simulink model "navigateObstacle_SF_solution"  (R2022a)
settings: Solver=ode23t  StartTime=0.0  StopTime=inf  RelTol=1e-3
InitFcn:
  | RPInit
model workspace (MAT data in the model file):
  mapForSim.obsMap = [0 0 0 0 0 0 0 0 0 0 0 0 ... (26600 elements, 133x200)]
  mapForSim.scaleFactor = 33.3333333333
  mapForSim.simMap = robotics.BinaryOccupancyGrid
  mapForSim.simMap.Grid = [1 1 1 1 1 1 1 1 1 1 1 1 ... (26600 elements, 133x200)]
  mapForSim.simMap.SharedProperties = matlabshared.autonomous.internal.SharedMapProperties
  mapForSim.simMap.SharedProperties.Resolution = 33.3333333333
  mapForSim.simMap.SharedProperties.GridSize = [133 200]
  mapForSim.simMap.SharedProperties.XLocalLimits = [0 6]
  mapForSim.simMap.SharedProperties.YLocalLimits = [0 3.99]
  mapForSim.simMap.SharedProperties.XWorldLimits = [0 6]
  mapForSim.simMap.SharedProperties.YWorldLimits = [0 3.99]
  mapForSim.simMap.SharedProperties.Width = 6
  mapForSim.simMap.SharedProperties.Height = 3.99
  mapForSim.simMap.SharedProperties.LocalOriginInWorldInternal = [0 0]
  mapForSim.simMap.LayerName = 'binaryLayer'
  mapForSim.simMap.Index = matlabshared.autonomous.internal.CircularBufferIndex
  mapForSim.simMap.Index.Head = [1 1]
  mapForSim.simMap.Index.Size = [133 200]
  mapForSim.simMap.Index.NewRegions = [0 0 0 0]
  mapForSim.simMap.Index.DropEntireMap = 0
  mapForSim.simMap.Index.DropTwoRegions = [0 0]
  mapForSim.simMap.Buffer = matlabshared.autonomous.internal.CircularBuffer
  mapForSim.simMap.Buffer.ConstVal = 0
  mapForSim.simMap.Buffer.DataType = 'logical'
  mapForSim.simMap.Buffer.Index = matlabshared.autonomous.internal.CircularBufferIndex
  mapForSim.simMap.Buffer.Index.Head = [1 1]
  mapForSim.simMap.Buffer.Index.Size = [133 200]
  mapForSim.simMap.Buffer.Index.NewRegions = [0 0 0 0]
  mapForSim.simMap.Buffer.Index.DropEntireMap = 0
  mapForSim.simMap.Buffer.Index.DropTwoRegions = [0 0]
  mapForSim.simMap.Buffer.Buffer = [1 1 1 1 1 1 1 1 1 1 1 1 ... (26600 elements, 133x200)]
  mapForSim.simMap.Buffer.BufferSize = [133 200 1]
  mapForSim.simMap.DefaultValueInternal = 0
  mapForSim.simMap.DataSize = [133 200]
  mapForSim.simMap.GridLocationInWorld = [0 0]
  mapForSim.simMap.GridOriginInLocal = [0 0]
  mapForSim.simMap.LocalOriginInWorld = [0 0]
  mapForSim.simMap.Resolution = 33.3333333333
  mapForSim.simMap.GridSize = [133 200]
  mapForSim.simMap.XLocalLimits = [0 6]
  mapForSim.simMap.YLocalLimits = [0 3.99]
  mapForSim.simMap.XWorldLimits = [0 6]
  mapForSim.simMap.YWorldLimits = [0 3.99]
  occGrid = robotics.BinaryOccupancyGrid
  occGrid.Grid = [1 1 1 1 1 1 1 1 1 1 1 1 ... (26600 elements, 133x200)]
  occGrid.SharedProperties = matlabshared.autonomous.internal.SharedMapProperties
  occGrid.SharedProperties.Resolution = 33.3333333333
  occGrid.SharedProperties.GridSize = [133 200]
  occGrid.SharedProperties.XLocalLimits = [0 6]
  occGrid.SharedProperties.YLocalLimits = [0 3.99]
  occGrid.SharedProperties.XWorldLimits = [0 6]
  occGrid.SharedProperties.YWorldLimits = [0 3.99]
  occGrid.SharedProperties.Width = 6
  occGrid.SharedProperties.Height = 3.99
  occGrid.SharedProperties.LocalOriginInWorldInternal = [0 0]
  occGrid.LayerName = 'binaryLayer'
  occGrid.Index = matlabshared.autonomous.internal.CircularBufferIndex
  occGrid.Index.Head = [1 1]
  occGrid.Index.Size = [133 200]
  occGrid.Index.NewRegions = [0 0 0 0]
  occGrid.Index.DropEntireMap = 0
  occGrid.Index.DropTwoRegions = [0 0]
  occGrid.Buffer = matlabshared.autonomous.internal.CircularBuffer
  occGrid.Buffer.ConstVal = 0
  occGrid.Buffer.DataType = 'logical'
  occGrid.Buffer.Index = matlabshared.autonomous.internal.CircularBufferIndex
  occGrid.Buffer.Index.Head = [1 1]
  occGrid.Buffer.Index.Size = [133 200]
  occGrid.Buffer.Index.NewRegions = [0 0 0 0]
  occGrid.Buffer.Index.DropEntireMap = 0
  occGrid.Buffer.Index.DropTwoRegions = [0 0]
  occGrid.Buffer.Buffer = [1 1 1 1 1 1 1 1 1 1 1 1 ... (26600 elements, 133x200)]
  occGrid.Buffer.BufferSize = [133 200 1]
  occGrid.DefaultValueInternal = 0
  occGrid.DataSize = [133 200]
  occGrid.GridLocationInWorld = [0 0]
  occGrid.GridOriginInLocal = [0 0]
  occGrid.LocalOriginInWorld = [0 0]
  occGrid.Resolution = 33.3333333333
  occGrid.GridSize = [133 200]
  occGrid.XLocalLimits = [0 6]
  occGrid.YLocalLimits = [0 3.99]
  occGrid.XWorldLimits = [0 6]
  occGrid.YWorldLimits = [0 3.99]
undefined symbols (not defined in the file): FloorSurface, Ref, RobotSurface, X, Y, Z
libraries: sm_lib x21, RP_Simulator_Components x12, nesl_utility x11, RoboticsPlayground x2
settings Model: Creator=josea  LastModifiedBy=josea
settings SolverCC: AlgebraicLoopSolver=TrustRegion
settings DataIOCC: ReturnWorkspaceOutputs=off
settings DebuggingCC: UnconnectedInputMsg=warning  UnconnectedOutputMsg=warning  SFMachineParentedDataDiag=warning  ArithmeticOperatorsInVariantConditions=warning
settings SFSimCC: SimUseLocalCustomCode=off  CustomCodeUndefinedFunction=UseInterfaceOnly
settings RTWCC: RTWUseLocalCustomCode=off
settings DiagnosticsConfigSet: SimMechanicsRigidlyBoundBlock=none
settings ExplorerConfigSet: InternalSimMechanicsExplorerSettings="<ExplorerConfiguration><canonicalview>default</canonicalview><AnimationSetting><BasePlaybackSpeed>1.0</BasePlaybackSpeed><PlaybackSpeedFactor>1.0</PlaybackSpeedFactor></AnimationSetting><TilePanel><TileInfo><Tiles Columns=\"1\" Count=\"1\" Rows=\"1\"><Column Weight=\"1\"/><Row Weight=\"1\"/><Tile Height=\"1\" Width=\"1\" X=\"0\" Y=\"0\"/></Tiles></TileInfo><SceneInfo><SceneViewer><BGColor><R>0.60000002384185791</R><G>0.60000002384185791</G><B>0.60000002384185791</B></BGColor><Camera><DoPerspective>off</DoPerspective><Position><X>1.02772841465426201</X><Y>-4.04307345472878321</Y><Z>5.44141009880599036</Z></Position><Center><X>1.02224964927968398</X><Y>0.073144029153633619</Y><Z>0.356451439525035663</Z></Center><Up><X>-0.0145298301603439817</X><Y>0.777168441982217129</Y><Z>0.629124865843375347</Z></Up><ViewLimDist>1</ViewLimDist><YLim>3.91326740754770297</YLim><XLim>6.08730485618531603</XLim></Camera></SceneViewer></SceneInfo></TilePanel><MechEditorPanel><Cameras/><GfxPanelCameraMap/><VideoCreator><PlaybackSpeedRatio>2.0</PlaybackSpeedRatio><FrameRate>30</FrameRate><VideoFormat>Motion JPEG AVI</VideoFormat><FrameSize>[1280 720]</FrameSize></VideoCreator></MechEditorPanel></ExplorerConfiguration>"

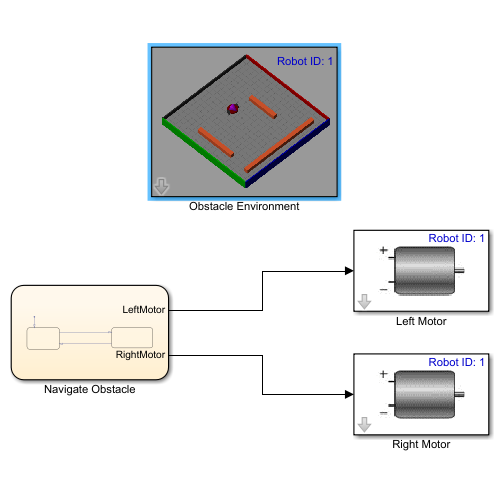
[thumbnail: Simulink's stored preview of the top-level diagram]
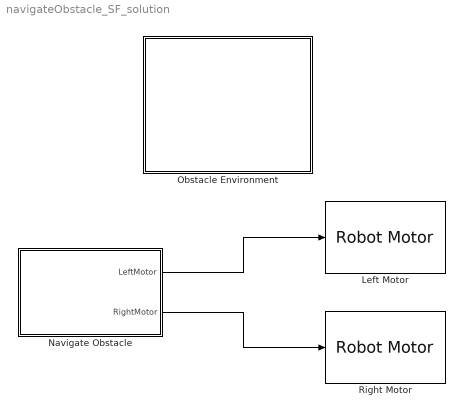
== system navigateObstacle_SF_solution ==
  Left Motor : RoboticsPlayground/Basic Sensors and Actuators/Robot Motor  robotId=1  motorChoice=1
      settings: SourceProductName=Robotics Playground
  Navigate Obstacle : Stateflow chart  TreatAsAtomicUnit=on
  Obstacle Environment : Subsystem  mask(RP Obstacle Environment){obs1=on, obsPose1=[0.054199    0.068864], obsWidth1=1.3052, obsLength1=1.156, obs2=off, obsPose2=[2.2548   -0.067351], obsWidth2=0.2899, obsLength2=3.4524, obs3=off, obsPose3=[-0.22694     -1.5652], obsWidth3=4.4627, obsLength3=0.4041, obs4=off, obsPose4=[-2.3001     0.17862], obsWidth4=0.4041, obsLength4=2.8726, obs5=off, obsPose5=[1.6535    -0.67545], obsWidth5=0.39824, obsLength5=0.71449, obs6=off, obsPose6=[3.1293     -1.6301], obsWidth6=0.60322, obsLength6=0.47438, obs7=off, obsPose7=[2 2], obsWidth7=0.8, obsLength7=0.4, obs8=off, obsPose8=[2 2], obsWidth8=0.8, obsLength8=0.4, obs9=off, obsPose9=[2 2], obsWidth9=0.8, obsLength9=0.4, obs10=off, obsPose10=[2 2], obsWidth10=0.8, obsLength10=0.4, arenaLength=6, arenaWidth=4, robotId=1, wheelBase=0.5, wheelRadius=0.1, robotColor=[0.5 0 0], startPose=[-1.2 -1.2]}
      mask prompts: obs1 "Enable"; obsPose1 "Position X Y [m]"; obsWidth1 "Width [m]"; obsLength1 "Length [m]"; obs2 "Enable"; obsPose2 "Position X Y [m]"; obsWidth2 "Width [m]"; obsLength2 "Length [m]"; obs3 "Enable"; obsPose3 "Position X Y [m]"; obsWidth3 "Width [m]"; obsLength3 "Length [m]"; obs4 "Enable"; obsPose4 "Position X Y [m]"; obsWidth4 "Width [m]"; obsLength4 "Length [m]"; obs5 "Enable"; obsPose5 "Position X Y [m]"; obsWidth5 "Width [m]"; obsLength5 "Length [m]"; obs6 "Enable"; obsPose6 "Position X Y [m]"; obsWidth6 "Width [m]"; obsLength6 "Length [m]"; obs7 "Enable"; obsPose7 "Position X Y [m]"; obsWidth7 "Width [m]"; obsLength7 "Length [m]"; obs8 "Enable"; obsPose8 "Position X Y [m]"; obsWidth8 "Width [m]"; obsLength8 "Length [m]"; obs9 "Enable"; obsPose9 "Position X Y [m]"; obsWidth9 "Width [m]"; obsLength9 "Length [m]"; obs10 "Enable"; obsPose10 "Position X Y [m]"; obsWidth10 "Width [m]"; obsLength10 "Length [m]"; arenaLength "Length [m]"; arenaWidth "Width [m]"; robotId "Robot ID"; wheelBase "Distance between wheels [m]"; wheelRadius "Wheel radius [m]"; robotColor "Color [R G B]"; startPose "Initial Position X Y [m]"
      mask help:
      | This block contains a virtual environment for a single robot to interact with walls, obstacles and objects. Sensors implemented in the Robotics Playground library can be used to obtain environment information and actuators to interact with the robot behavior.
      |
      | Motor mapping for the robot is as follows:
      |
      | Motor 1 -> Left wheel motor torque
      | Motor 2 -> Right wheel motor torque
      settings: CopyFcn=|
      | set_param(gcs,'InitFcn','RPInit');
      | set_param(gcs,'Solver','ode23t');
      | set_param(gcs, 'EnablePacing', 'on')
      | set_param(gcs, 'PacingRate', 1)
      mask Help: web('obstacle_arena.htm')
      mask Callback obs1: commentObstacles(gcb)
      mask Callback obs2: commentObstacles(gcb)
      mask Callback obs3: commentObstacles(gcb)
      mask Callback obs4: commentObstacles(gcb)
      mask Callback obs5: commentObstacles(gcb)
      mask Callback obs6: commentObstacles(gcb)
      mask Callback obs7: commentObstacles(gcb)
      mask Callback obs8: commentObstacles(gcb)
      mask Callback obs9: commentObstacles(gcb)
      mask Callback obs10: commentObstacles(gcb)
      mask DialogControl obsT Prompt: Obstacle settings
      mask DialogControl Container19 Prompt: Set Obstacles Interactively
      mask DialogControl Control2 Prompt: Set Obstacles
      mask DialogControl Control2 Callback: setObstaclesUI(gcb)
      mask DialogControl Control3 Prompt: Disable all obstacles
      mask DialogControl Control3 Callback: disableObstacles(gcb)
      mask DialogControl Container21 Prompt: Obstacle Details
      mask DialogControl obsc1 Prompt: Obstacle 1
      mask DialogControl obsc2 Prompt: Obstacle 2
      mask DialogControl obsc3 Prompt: Obstacle 3
      mask DialogControl obsc4 Prompt: Obstacle 4
      mask DialogControl obsc5 Prompt: Obstacle 5
      mask DialogControl obsc6 Prompt: Obstacle 6
      mask DialogControl obsc7 Prompt: Obstacle 7
      mask DialogControl obsc8 Prompt: Obstacle 8
      mask DialogControl obsc9 Prompt: Obstacle 9
      mask DialogControl obsc10 Prompt: Obstacle 10
      mask DialogControl Container6 Prompt: Arena settings
      mask DialogControl Container4 Prompt: Robot settings
      mask Display:
      | color('white');
      | plot([100,100,100,100]*1,[100,100,100,100]*1);
      | plot([100,100,100,100]*0,[100,100,100,100]*0);
      | image('ObstacleEnv.PNG')
      | color('blue');
      | id=eval(get_param(gcb,'robotId'));
      | text(99, 92, ['Robot ID: ' num2str(id)], 'horizontalAlignment', 'right');
  Right Motor : RoboticsPlayground/Basic Sensors and Actuators/Robot Motor  robotId=1  motorChoice=2
      settings: SourceProductName=Robotics Playground
  wires:
  Navigate Obstacle/1(LeftMotor) -> Left Motor/1
  Navigate Obstacle/2(RightMotor) -> Right Motor/1

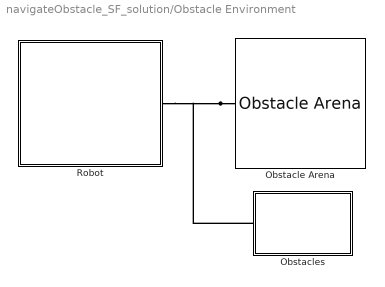
== system navigateObstacle_SF_solution/Obstacle Environment ==
  Obstacle Arena : RP_Simulator_Components/Obstacle Arena  length=arenaLength  width=arenaWidth  robotRadius=wheelBase/2
  Obstacles : Subsystem
  Robot : Subsystem  AncestorBlock=RP_Simulator_Components/Contact Tank Robot  mask(RP Contact Tank Robot){robotId=robotId, wheelRadius=wheelRadius, wheelBase=wheelBase, wheelThickness=0.025, chassisThickness=0.05, startPose=startPose, choice=off, sensorTs=0.05, wheelMass=0.2, chassisMass=0.5, maxWheelTorque=1, floorSize=[arenaLength arenaWidth], wheelColor=[0.25 0.25 0.25], chassisColor=robotColor}
      mask prompts: robotId "Robot ID"; wheelRadius "Wheel Radius [m]"; wheelBase "Wheelbase [m]"; wheelThickness "Wheel Thickness [m]"; chassisThickness "Chassis Thickness [m]"; startPose "Start Position [m]"; choice "Reverse Start Position"; sensorTs "Sensor sample time [s]"; wheelMass "Wheel Mass [kg]"; chassisMass "Chassis Mass [kg]"; maxWheelTorque "Maximum wheel torque [N*m]"; floorSize "Floor Dimensions [m]"; wheelColor "Wheel Color"; chassisColor "Chassis Color"
      mask help:
      | This robot implements contact between the robot wheels and the floor of an arena. The stck-slip friction implemented using contact force libraries makes the robot behavior more realistic. The inputs to the robot are now motor torque, which is set using the Robotics Playground Motor blocks. The motor mappings are as follows:
      |
      | Motor 1 -> Left wheel motor torque
      | Motor 2 -> Right wheel motor torque
      mask init:
      | block=gcb;
      | ID=num2str(eval(get_param(block,'robotId')));
      | 
      | set_param([block '/motor1t'],'GotoTag',['R' ID 'motor1t']);
      | set_param([block '/motor2t'],'GotoTag',['R' ID 'motor2t']);
      | set_param([block '/motor1q'],'GotoTag',['R' ID 'motor1q']);
      | set_param([block '/motor1w'],'GotoTag',['R' ID 'motor1w']);
      | set_param([block '/motor2q'],'GotoTag',['R' ID 'motor2q']);
      | set_param([block '/motor2w'],'GotoTag',['R' ID 'motor2w']);
      | set_param([block '/xPose'],'GotoTag',['R' ID 'xPose']);
      | set_param([block '/yPose'],'GotoTag',['R' ID 'yPose']);
      | set_param([block '/tPose'],'GotoTag',['R' ID 'tPose']);
      | set_param([block '/tRate'],'GotoTag',['R' ID 'tRate']);
      | set_param([block '/tAngle'],'GotoTag',['R' ID 'tAngle']);
      | 
      | % Add sensor visuals
      | 
      | addSensors(block,eval(ID));
      mask DialogControl KinContainer Prompt: Kinematics
      mask DialogControl DynamicsContainer Prompt: Dynamics
      mask DialogControl AppearanceContainer Prompt: Appearance
      mask Display:
      | image('discRobot.PNG')
      | port_label('Rconn',1,'RP-Bus')
  connections:
  Obstacle Arena/LConn1 -- Obstacles/LConn1 -- Robot/RConn1

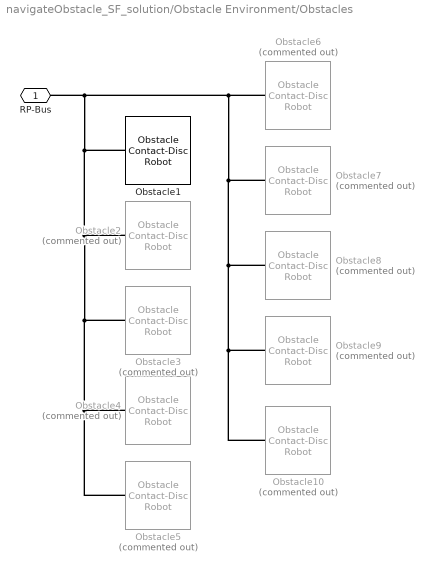
== system navigateObstacle_SF_solution/Obstacle Environment/Obstacles ==
  Obstacle1 : RP_Simulator_Components/Obstacle Contact-Disc Robot  Pose=obsPose1  width=obsWidth1  length=obsLength1  height=0.3  color=[1.0 0.4 0.2]
  Obstacle10 : RP_Simulator_Components/Obstacle Contact-Disc Robot  Commented=on  Pose=obsPose10  width=obsWidth10  length=obsLength10  height=0.3  color=[1.0 0.4 0.2]
  Obstacle2 : RP_Simulator_Components/Obstacle Contact-Disc Robot  Commented=on  Pose=obsPose2  width=obsWidth2  length=obsLength2  height=0.3  color=[1.0 0.4 0.2]
  Obstacle3 : RP_Simulator_Components/Obstacle Contact-Disc Robot  Commented=on  Pose=obsPose3  width=obsWidth3  length=obsLength3  height=0.3  color=[1.0 0.4 0.2]
  Obstacle4 : RP_Simulator_Components/Obstacle Contact-Disc Robot  Commented=on  Pose=obsPose4  width=obsWidth4  length=obsLength4  height=0.3  color=[1.0 0.4 0.2]
  Obstacle5 : RP_Simulator_Components/Obstacle Contact-Disc Robot  Commented=on  Pose=obsPose5  width=obsWidth5  length=obsLength5  height=0.3  color=[1.0 0.4 0.2]
  Obstacle6 : RP_Simulator_Components/Obstacle Contact-Disc Robot  Commented=on  Pose=obsPose6  width=obsWidth6  length=obsLength6  height=0.3  color=[1.0 0.4 0.2]
  Obstacle7 : RP_Simulator_Components/Obstacle Contact-Disc Robot  Commented=on  Pose=obsPose7  width=obsWidth7  length=obsLength7  height=0.3  color=[1.0 0.4 0.2]
  Obstacle8 : RP_Simulator_Components/Obstacle Contact-Disc Robot  Commented=on  Pose=obsPose8  width=obsWidth8  length=obsLength8  height=0.3  color=[1.0 0.4 0.2]
  Obstacle9 : RP_Simulator_Components/Obstacle Contact-Disc Robot  Commented=on  Pose=obsPose9  width=obsWidth9  length=obsLength9  height=0.3  color=[1.0 0.4 0.2]
  RP-Bus : PMIOPort  Side=Left
  connections:
  Obstacle1/LConn1 -- Obstacle5/LConn1 -- Obstacle4/LConn1 -- Obstacle3/LConn1 -- Obstacle2/LConn1 -- Obstacle6/LConn1 -- Obstacle10/LConn1 -- Obstacle9/LConn1 -- Obstacle8/LConn1 -- Obstacle7/LConn1 -- RP-Bus/RConn1

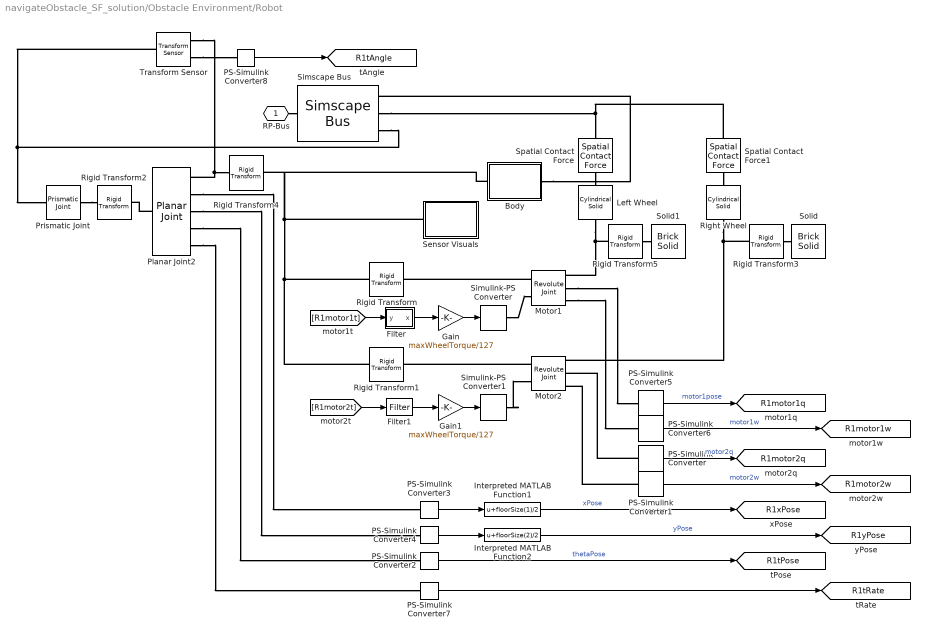
== system navigateObstacle_SF_solution/Obstacle Environment/Robot ==
  Body : Subsystem
  Filter : Subsystem
  Filter1 : RP_Simulator_Components/Contact Tank Robot/Filter  SystemSampleTime=-1  VariantActivationTime=update diagram  Latency=0  AutoFrameSizeCalculation=off
  Gain : Gain  Gain=maxWheelTorque/127
  Gain1 : Gain  Gain=maxWheelTorque/127
  Interpreted MATLAB Function1 : MATLABFcn  MATLABFcn=u+floorSize(1)/2
  Interpreted MATLAB Function2 : MATLABFcn  MATLABFcn=u+floorSize(2)/2
  Left Wheel : sm_lib/Body Elements/Cylindrical Solid  GraphicAmbientColor=[0.15 0.15 0.15 1.0]  BasedOnType=Mass  CenterOfMass=[0 0 0]  CenterOfMassUnits=m  GraphicDiffuseColor=wheelColor  CylinderLength=wheelThickness  CylinderLengthUnits=m  CylinderRadius=wheelRadius  CylinderRadiusUnits=m  Density=1000  DensityUnits=kg/m^3  DoExposeReferenceFrame=on  GraphicEmissiveColor=[0.0 0.0 0.0 1.0]  ExportEntireGeometry=on  SerializedFrames=<Frames/>  MarkerShape=Sphere  MarkerSize=10  GraphicType=FromGeometry  InertiaType=CalculateFromGeometry  Mass=wheelMass  MassUnits=kg  MomentsOfInertia=[1 1 1]  MomentsOfInertiaUnits=kg*m^2  GraphicOpacity=1.0  ProductsOfInertia=[1 1 1]  ProductsOfInertiaUnits=kg*m^2  GraphicShininess=75  GraphicSpecularColor=[0.5 0.5 0.5 1.0]  GraphicVisPropType=SimpleVisualProperties
  Motor1 : sm_lib/Joints/Revolute Joint  JointMode=Normal  SenseConstraintForce=off  SenseConstraintForceX=off  SenseConstraintForceY=off  SenseConstraintForceZ=off  SenseConstraintTorque=off  SenseConstraintTorqueX=off  SenseConstraintTorqueY=off  SenseConstraintTorqueZ=off  SenseTotalForce=off  SenseTotalForceX=off  SenseTotalForceY=off  SenseTotalForceZ=off  SenseTotalTorque=off  SenseTotalTorqueX=off  SenseTotalTorqueY=off  SenseTotalTorqueZ=off  CompositeWrenchDir=FollowerOnBase  CompositeWrenchFrame=BaseFrame  EquilibriumPosition=0  EquilibriumPositionUnits=deg  SpringStiffness=0  SpringStiffnessUnits=N*m/deg  DampingCoefficient=0.004  DampingCoefficientUnits=N*m/(deg/s)  TorqueActuationMode=InputTorque  MotionActuationMode=ComputedMotion  SensePosition=on  SenseVelocity=on  SenseAcceleration=off  SenseTorqueForce=off  SenseLowerLimitTorqueForce=off  SenseUpperLimitTorqueForce=off  LowerLimitSpecify=off  LowerLimitBound=-90  LowerLimitBoundUnits=deg  LowerLimitStiffness=1e4  LowerLimitStiffnessUnits=N*m/deg  LowerLimitDamping=10  LowerLimitDampingUnits=N*m/(deg/s)  LowerLimitTransitionRegionWidth=0.1  LowerLimitTransitionRegionWidthUnits=deg  UpperLimitSpecify=off  UpperLimitBound=90  UpperLimitBoundUnits=deg  UpperLimitStiffness=1e4  UpperLimitStiffnessUnits=N*m/deg  UpperLimitDamping=10  UpperLimitDampingUnits=N*m/(deg/s)  UpperLimitTransitionRegionWidth=0.1  UpperLimitTransitionRegionWidthUnits=deg  PositionTargetSpecify=off  PositionTargetPriority=High  PositionTargetValue=0  PositionTargetValueUnits=deg  VelocityTargetSpecify=off  VelocityTargetPriority=High  VelocityTargetValue=0  VelocityTargetValueUnits=deg/s
  Motor2 : sm_lib/Joints/Revolute Joint  JointMode=Normal  SenseConstraintForce=off  SenseConstraintForceX=off  SenseConstraintForceY=off  SenseConstraintForceZ=off  SenseConstraintTorque=off  SenseConstraintTorqueX=off  SenseConstraintTorqueY=off  SenseConstraintTorqueZ=off  SenseTotalForce=off  SenseTotalForceX=off  SenseTotalForceY=off  SenseTotalForceZ=off  SenseTotalTorque=off  SenseTotalTorqueX=off  SenseTotalTorqueY=off  SenseTotalTorqueZ=off  CompositeWrenchDir=FollowerOnBase  CompositeWrenchFrame=BaseFrame  EquilibriumPosition=0  EquilibriumPositionUnits=deg  SpringStiffness=0  SpringStiffnessUnits=N*m/deg  DampingCoefficient=0.004  DampingCoefficientUnits=N*m/(deg/s)  TorqueActuationMode=InputTorque  MotionActuationMode=ComputedMotion  SensePosition=on  SenseVelocity=on  SenseAcceleration=off  SenseTorqueForce=off  SenseLowerLimitTorqueForce=off  SenseUpperLimitTorqueForce=off  LowerLimitSpecify=off  LowerLimitBound=-90  LowerLimitBoundUnits=deg  LowerLimitStiffness=1e4  LowerLimitStiffnessUnits=N*m/deg  LowerLimitDamping=10  LowerLimitDampingUnits=N*m/(deg/s)  LowerLimitTransitionRegionWidth=0.1  LowerLimitTransitionRegionWidthUnits=deg  UpperLimitSpecify=off  UpperLimitBound=90  UpperLimitBoundUnits=deg  UpperLimitStiffness=1e4  UpperLimitStiffnessUnits=N*m/deg  UpperLimitDamping=10  UpperLimitDampingUnits=N*m/(deg/s)  UpperLimitTransitionRegionWidth=0.1  UpperLimitTransitionRegionWidthUnits=deg  PositionTargetSpecify=off  PositionTargetPriority=High  PositionTargetValue=0  PositionTargetValueUnits=deg  VelocityTargetSpecify=off  VelocityTargetPriority=High  VelocityTargetValue=0  VelocityTargetValueUnits=deg/s
  PS-Simulink Converter{,1,3..6} (6 alike) : nesl_utility/PS-Simulink Converter  PhysicalDomain=network_engine_domain  SubClassName=ps_output  LeftPortType=input  RightPortType=output  PseudoPeriodic=off  Frequencies=[]  VectorFormat=1-D array  Unit=1  AffineConversion=off
      settings: SourceProductBaseCode=SS,PW,VE
  PS-Simulink Converter2 : nesl_utility/PS-Simulink Converter  PhysicalDomain=network_engine_domain  SubClassName=ps_output  LeftPortType=input  RightPortType=output  PseudoPeriodic=off  Frequencies=[]  VectorFormat=1-D array  Unit=rad  AffineConversion=off
      settings: SourceProductBaseCode=SS,PW,VE
  PS-Simulink Converter7 : nesl_utility/PS-Simulink Converter  PhysicalDomain=network_engine_domain  SubClassName=ps_output  LeftPortType=input  RightPortType=output  PseudoPeriodic=off  Frequencies=[]  VectorFormat=1-D array  Unit=deg/s  AffineConversion=off
      settings: SourceProductBaseCode=SS,PW,VE
  PS-Simulink Converter8 : nesl_utility/PS-Simulink Converter  PhysicalDomain=network_engine_domain  SubClassName=ps_output  LeftPortType=input  RightPortType=output  PseudoPeriodic=off  Frequencies=[]  VectorFormat=1-D array  Unit=deg  AffineConversion=off
      settings: SourceProductBaseCode=SS,PW,VE
  Planar Joint2 : sm_lib/Joints/Planar Joint  JointMode=Normal  SenseConstraintForce=off  SenseConstraintForceX=off  SenseConstraintForceY=off  SenseConstraintForceZ=off  SenseConstraintTorque=off  SenseConstraintTorqueX=off  SenseConstraintTorqueY=off  SenseConstraintTorqueZ=off  SenseTotalForce=off  SenseTotalForceX=off  SenseTotalForceY=off  SenseTotalForceZ=off  SenseTotalTorque=off  SenseTotalTorqueX=off  SenseTotalTorqueY=off  SenseTotalTorqueZ=off  CompositeWrenchDir=FollowerOnBase  CompositeWrenchFrame=BaseFrame  PxEquilibriumPosition=0  PxEquilibriumPositionUnits=m  PxSpringStiffness=0  PxSpringStiffnessUnits=N/m  PxDampingCoefficient=5  PxDampingCoefficientUnits=N/(m/s)  PxTorqueActuationMode=NoTorque  PxMotionActuationMode=ComputedMotion  PxSensePosition=on  PxSenseVelocity=off  PxSenseAcceleration=off  PxSenseTorqueForce=off  PxSenseLowerLimitTorqueForce=off  PxSenseUpperLimitTorqueForce=off  PxLowerLimitSpecify=off  PxLowerLimitBound=-1  PxLowerLimitBoundUnits=m  PxLowerLimitStiffness=1e6  PxLowerLimitStiffnessUnits=N/m  PxLowerLimitDamping=1e3  PxLowerLimitDampingUnits=N/(m/s)  PxLowerLimitTransitionRegionWidth=1e-4  PxLowerLimitTransitionRegionWidthUnits=m  PxUpperLimitSpecify=off  PxUpperLimitBound=1  PxUpperLimitBoundUnits=m  PxUpperLimitStiffness=1e6  PxUpperLimitStiffnessUnits=N/m  PxUpperLimitDamping=1e3  PxUpperLimitDampingUnits=N/(m/s)  PxUpperLimitTransitionRegionWidth=1e-4  PxUpperLimitTransitionRegionWidthUnits=m  PxPositionTargetSpecify=on  PxPositionTargetPriority=High  PxPositionTargetValue=startPose(1)  PxPositionTargetValueUnits=m  PxVelocityTargetSpecify=off  PxVelocityTargetPriority=High  PxVelocityTargetValue=0  PxVelocityTargetValueUnits=m/s  PyEquilibriumPosition=0  PyEquilibriumPositionUnits=m  PySpringStiffness=0  PySpringStiffnessUnits=N/m  PyDampingCoefficient=5  PyDampingCoefficientUnits=N/(m/s)  PyTorqueActuationMode=NoTorque  PyMotionActuationMode=ComputedMotion  PySensePosition=on  PySenseVelocity=off  PySenseAcceleration=off  PySenseTorqueForce=off  PySenseLowerLimitTorqueForce=off  PySenseUpperLimitTorqueForce=off  PyLowerLimitSpecify=off  PyLowerLimitBound=-1  PyLowerLimitBoundUnits=m  PyLowerLimitStiffness=1e6  PyLowerLimitStiffnessUnits=N/m  PyLowerLimitDamping=1e3  PyLowerLimitDampingUnits=N/(m/s)  PyLowerLimitTransitionRegionWidth=1e-4  PyLowerLimitTransitionRegionWidthUnits=m  PyUpperLimitSpecify=off  PyUpperLimitBound=1  PyUpperLimitBoundUnits=m  PyUpperLimitStiffness=1e6  PyUpperLimitStiffnessUnits=N/m  PyUpperLimitDamping=1e3  PyUpperLimitDampingUnits=N/(m/s)  PyUpperLimitTransitionRegionWidth=1e-4  PyUpperLimitTransitionRegionWidthUnits=m  PyPositionTargetSpecify=on  PyPositionTargetPriority=High  PyPositionTargetValue=startPose(2)  PyPositionTargetValueUnits=m  PyVelocityTargetSpecify=off  PyVelocityTargetPriority=High  PyVelocityTargetValue=0  PyVelocityTargetValueUnits=m/s  RzEquilibriumPosition=0  RzEquilibriumPositionUnits=deg  RzSpringStiffness=0  RzSpringStiffnessUnits=N*m/deg  RzDampingCoefficient=2/45  RzDampingCoefficientUnits=N*m/(deg/s)  RzTorqueActuationMode=NoTorque  RzMotionActuationMode=ComputedMotion  RzSensePosition=on  RzSenseVelocity=on  RzSenseAcceleration=off  RzSenseTorqueForce=off  RzSenseLowerLimitTorqueForce=off  RzSenseUpperLimitTorqueForce=off  RzLowerLimitSpecify=off  RzLowerLimitBound=-90  RzLowerLimitBoundUnits=deg  RzLowerLimitStiffness=1e4  RzLowerLimitStiffnessUnits=N*m/deg  RzLowerLimitDamping=10  RzLowerLimitDampingUnits=N*m/(deg/s)  RzLowerLimitTransitionRegionWidth=0.1  RzLowerLimitTransitionRegionWidthUnits=deg  RzUpperLimitSpecify=off  RzUpperLimitBound=90  RzUpperLimitBoundUnits=deg  RzUpperLimitStiffness=1e4  RzUpperLimitStiffnessUnits=N*m/deg  RzUpperLimitDamping=10  RzUpperLimitDampingUnits=N*m/(deg/s)  RzUpperLimitTransitionRegionWidth=0.1  RzUpperLimitTransitionRegionWidthUnits=deg  RzPositionTargetSpecify=off  RzPositionTargetPriority=High  RzPositionTargetValue=0  RzPositionTargetValueUnits=deg  RzVelocityTargetSpecify=off  RzVelocityTargetPriority=High  RzVelocityTargetValue=0  RzVelocityTargetValueUnits=deg/s
  Prismatic Joint : sm_lib/Joints/Prismatic Joint  JointMode=Normal  SenseConstraintForce=off  SenseConstraintForceX=off  SenseConstraintForceY=off  SenseConstraintForceZ=off  SenseConstraintTorque=off  SenseConstraintTorqueX=off  SenseConstraintTorqueY=off  SenseConstraintTorqueZ=off  SenseTotalForce=off  SenseTotalForceX=off  SenseTotalForceY=off  SenseTotalForceZ=off  SenseTotalTorque=off  SenseTotalTorqueX=off  SenseTotalTorqueY=off  SenseTotalTorqueZ=off  CompositeWrenchDir=FollowerOnBase  CompositeWrenchFrame=BaseFrame  EquilibriumPosition=0  EquilibriumPositionUnits=m  SpringStiffness=0  SpringStiffnessUnits=N/m  DampingCoefficient=0  DampingCoefficientUnits=N/(m/s)  TorqueActuationMode=NoTorque  MotionActuationMode=ComputedMotion  SensePosition=off  SenseVelocity=off  SenseAcceleration=off  SenseTorqueForce=off  SenseLowerLimitTorqueForce=off  SenseUpperLimitTorqueForce=off  LowerLimitSpecify=off  LowerLimitBound=-1  LowerLimitBoundUnits=m  LowerLimitStiffness=1e6  LowerLimitStiffnessUnits=N/m  LowerLimitDamping=1e3  LowerLimitDampingUnits=N/(m/s)  LowerLimitTransitionRegionWidth=1e-4  LowerLimitTransitionRegionWidthUnits=m  UpperLimitSpecify=off  UpperLimitBound=1  UpperLimitBoundUnits=m  UpperLimitStiffness=1e6  UpperLimitStiffnessUnits=N/m  UpperLimitDamping=1e3  UpperLimitDampingUnits=N/(m/s)  UpperLimitTransitionRegionWidth=1e-4  UpperLimitTransitionRegionWidthUnits=m  PositionTargetSpecify=on  PositionTargetPriority=High  PositionTargetValue=0.02  PositionTargetValueUnits=m  VelocityTargetSpecify=off  VelocityTargetPriority=High  VelocityTargetValue=0  VelocityTargetValueUnits=m/s
  Right Wheel : sm_lib/Body Elements/Cylindrical Solid  GraphicAmbientColor=[0.15 0.15 0.15 1.0]  BasedOnType=Mass  CenterOfMass=[0 0 0]  CenterOfMassUnits=m  GraphicDiffuseColor=wheelColor  CylinderLength=wheelThickness  CylinderLengthUnits=m  CylinderRadius=wheelRadius  CylinderRadiusUnits=m  Density=1000  DensityUnits=kg/m^3  DoExposeReferenceFrame=on  GraphicEmissiveColor=[0.0 0.0 0.0 1.0]  ExportEntireGeometry=on  SerializedFrames=<Frames/>  MarkerShape=Sphere  MarkerSize=10  GraphicType=FromGeometry  InertiaType=CalculateFromGeometry  Mass=wheelMass  MassUnits=kg  MomentsOfInertia=[1 1 1]  MomentsOfInertiaUnits=kg*m^2  GraphicOpacity=1.0  ProductsOfInertia=[1 1 1]  ProductsOfInertiaUnits=kg*m^2  GraphicShininess=75  GraphicSpecularColor=[0.5 0.5 0.5 1.0]  GraphicVisPropType=SimpleVisualProperties
  Rigid Transform : sm_lib/Frames and Transforms/Rigid Transform  TranslationMethod=StandardAxis  TranslationStandardOffset=wheelBase/2  TranslationLengthUnit=m  TranslationStandardAxis=+Y  TranslationCartesianOffset=[0 0 0]  TranslationROffset=0  TranslationROffsetUnits=m  TranslationZOffset=0  TranslationZOffsetUnits=m  TranslationThetaOffset=0  TranslationThetaOffsetUnits=deg  RotationMethod=AlignedAxes  RotationAngleUnits=deg  RotationStandardAxis=+Z  RotationAngle=0.0  RotationArbitraryAxis=[0 0 1]  FollAlignAxisA=+Z  BaseAlignAxisA=+Y  FollAlignAxisB=+X  BaseAlignAxisB=+X  RotationSequenceAxes=FollowerAxes  RotationSequence=XYX  RotationSequenceAngles=[0 0 0]  RotationSequenceAnglesUnits=deg  RotationMatrix=[1 0 0; 0 1 0; 0 0 1]
  Rigid Transform1 : sm_lib/Frames and Transforms/Rigid Transform  TranslationMethod=StandardAxis  TranslationStandardOffset=wheelBase/2  TranslationLengthUnit=m  TranslationStandardAxis=-Y  TranslationCartesianOffset=[0 0 0]  TranslationROffset=0  TranslationROffsetUnits=m  TranslationZOffset=0  TranslationZOffsetUnits=m  TranslationThetaOffset=0  TranslationThetaOffsetUnits=deg  RotationMethod=AlignedAxes  RotationAngleUnits=deg  RotationStandardAxis=+Z  RotationAngle=0.0  RotationArbitraryAxis=[0 0 1]  FollAlignAxisA=+Z  BaseAlignAxisA=+Y  FollAlignAxisB=+X  BaseAlignAxisB=+X  RotationSequenceAxes=FollowerAxes  RotationSequence=XYX  RotationSequenceAngles=[0 0 0]  RotationSequenceAnglesUnits=deg  RotationMatrix=[1 0 0; 0 1 0; 0 0 1]
  Rigid Transform2 : sm_lib/Frames and Transforms/Rigid Transform  TranslationMethod=StandardAxis  TranslationStandardOffset=wheelRadius  TranslationLengthUnit=m  TranslationStandardAxis=+Z  TranslationCartesianOffset=[0 0 0]  TranslationROffset=0  TranslationROffsetUnits=m  TranslationZOffset=0  TranslationZOffsetUnits=m  TranslationThetaOffset=0  TranslationThetaOffsetUnits=deg  RotationMethod=None  RotationAngleUnits=deg  RotationStandardAxis=+Z  RotationAngle=0.0  RotationArbitraryAxis=[0 0 1]  FollAlignAxisA=+Z  BaseAlignAxisA=+Y  FollAlignAxisB=+X  BaseAlignAxisB=+X  RotationSequenceAxes=FollowerAxes  RotationSequence=XYX  RotationSequenceAngles=[0 0 0]  RotationSequenceAnglesUnits=deg  RotationMatrix=[1 0 0; 0 1 0; 0 0 1]
  Rigid Transform3 : sm_lib/Frames and Transforms/Rigid Transform  TranslationMethod=Cartesian  TranslationStandardOffset=0  TranslationLengthUnit=m  TranslationStandardAxis=+Z  TranslationCartesianOffset=[wheelRadius/2 0 0]  TranslationROffset=0  TranslationROffsetUnits=m  TranslationZOffset=0  TranslationZOffsetUnits=m  TranslationThetaOffset=0  TranslationThetaOffsetUnits=deg  RotationMethod=None  RotationAngleUnits=deg  RotationStandardAxis=+Z  RotationAngle=0.0  RotationArbitraryAxis=[0 0 1]  FollAlignAxisA=+X  BaseAlignAxisA=+Y  FollAlignAxisB=+Y  BaseAlignAxisB=+Z  RotationSequenceAxes=FollowerAxes  RotationSequence=XYX  RotationSequenceAngles=[0 0 0]  RotationSequenceAnglesUnits=deg  RotationMatrix=[1 0 0; 0 1 0; 0 0 1]
  Rigid Transform4 : sm_lib/Frames and Transforms/Rigid Transform  TranslationMethod=None  TranslationStandardOffset=0  TranslationLengthUnit=m  TranslationStandardAxis=+Z  TranslationCartesianOffset=[0 0 0]  TranslationROffset=0  TranslationROffsetUnits=m  TranslationZOffset=0  TranslationZOffsetUnits=m  TranslationThetaOffset=0  TranslationThetaOffsetUnits=deg  RotationMethod=StandardAxis  RotationAngleUnits=deg  RotationStandardAxis=+Z  RotationAngle=180*choice  RotationArbitraryAxis=[0 0 1]  FollAlignAxisA=+X  BaseAlignAxisA=+Y  FollAlignAxisB=+Y  BaseAlignAxisB=+Z  RotationSequenceAxes=FollowerAxes  RotationSequence=XYX  RotationSequenceAngles=[0 0 0]  RotationSequenceAnglesUnits=deg  RotationMatrix=[1 0 0; 0 1 0; 0 0 1]
  Rigid Transform5 : sm_lib/Frames and Transforms/Rigid Transform  TranslationMethod=Cartesian  TranslationStandardOffset=0  TranslationLengthUnit=m  TranslationStandardAxis=+Z  TranslationCartesianOffset=[wheelRadius/2 0 0]  TranslationROffset=0  TranslationROffsetUnits=m  TranslationZOffset=0  TranslationZOffsetUnits=m  TranslationThetaOffset=0  TranslationThetaOffsetUnits=deg  RotationMethod=None  RotationAngleUnits=deg  RotationStandardAxis=+Z  RotationAngle=0.0  RotationArbitraryAxis=[0 0 1]  FollAlignAxisA=+X  BaseAlignAxisA=+Y  FollAlignAxisB=+Y  BaseAlignAxisB=+Z  RotationSequenceAxes=FollowerAxes  RotationSequence=XYX  RotationSequenceAngles=[0 0 0]  RotationSequenceAnglesUnits=deg  RotationMatrix=[1 0 0; 0 1 0; 0 0 1]
  Sensor Visuals : Subsystem
  Simscape Bus : SimscapeBus  HierarchyStrings=RobotSurface;FloorSurface;Ref
  Simulink-PS Converter : nesl_utility/Simulink-PS Converter  PhysicalDomain=network_engine_domain  SubClassName=ps_input  LeftPortType=input  RightPortType=output  PseudoPeriodic=off  Frequencies=[]  NoiseDistribution=none  NoiseParameters=[]  Unit=1  AffineConversion=off  FilteringAndDerivatives=provide  SimscapeFilterOrder=1  InputFilterTimeConstant=0.05  UdotUserProvided=0
      settings: SourceProductBaseCode=SS,PW,VE
  Simulink-PS Converter1 : nesl_utility/Simulink-PS Converter  PhysicalDomain=network_engine_domain  SubClassName=ps_input  LeftPortType=input  RightPortType=output  PseudoPeriodic=off  Frequencies=[]  NoiseDistribution=none  NoiseParameters=[]  Unit=1  AffineConversion=off  FilteringAndDerivatives=provide  SimscapeFilterOrder=1  InputFilterTimeConstant=0.05  UdotUserProvided=0
      settings: SourceProductBaseCode=SS,PW,VE
  Solid : sm_lib/Body Elements/Brick Solid  GraphicAmbientColor=[0.15 0.15 0.15 1.0]  BasedOnType=Density  BrickDimensions=[wheelRadius*0.8 wheelThickness*1.05 wheelThickness*1.05]  BrickDimensionUnits=m  CenterOfMass=[0 0 0]  CenterOfMassUnits=m  GraphicDiffuseColor=[0.0 0.8 0.8]  Density=1000  DensityUnits=kg/m^3  DoExposeReferenceFrame=on  GraphicEmissiveColor=[0.0 0.0 0.0 1.0]  ExportEntireGeometry=off  SerializedFrames=<Frames/>  MarkerShape=Sphere  MarkerSize=10  GraphicType=FromGeometry  InertiaType=CalculateFromGeometry  Mass=1  MassUnits=kg  MomentsOfInertia=[1 1 1]  MomentsOfInertiaUnits=kg*m^2  GraphicOpacity=1.0  ProductsOfInertia=[1 1 1]  ProductsOfInertiaUnits=kg*m^2  GraphicShininess=75  GraphicSpecularColor=[0.5 0.5 0.5 1.0]  GraphicVisPropType=SimpleVisualProperties
  Solid1 : sm_lib/Body Elements/Brick Solid  GraphicAmbientColor=[0.15 0.15 0.15 1.0]  BasedOnType=Density  BrickDimensions=[wheelRadius*0.8 wheelThickness*1.05 wheelThickness*1.05]  BrickDimensionUnits=m  CenterOfMass=[0 0 0]  CenterOfMassUnits=m  GraphicDiffuseColor=[0.0 0.8 0.8]  Density=1000  DensityUnits=kg/m^3  DoExposeReferenceFrame=on  GraphicEmissiveColor=[0.0 0.0 0.0 1.0]  ExportEntireGeometry=off  SerializedFrames=<Frames/>  MarkerShape=Sphere  MarkerSize=10  GraphicType=FromGeometry  InertiaType=CalculateFromGeometry  Mass=1  MassUnits=kg  MomentsOfInertia=[1 1 1]  MomentsOfInertiaUnits=kg*m^2  GraphicOpacity=1.0  ProductsOfInertia=[1 1 1]  ProductsOfInertiaUnits=kg*m^2  GraphicShininess=75  GraphicSpecularColor=[0.5 0.5 0.5 1.0]  GraphicVisPropType=SimpleVisualProperties
  Spatial Contact Force : sm_lib/Forces and Torques/Spatial Contact Force  SenseContactBaseRotation=off  SenseContactBaseTranslation=off  CoefficientOfDynamicFriction=0.5  CoefficientOfStaticFriction=0.7  NormalDamping=1e2  NormalDampingUnits=N/(m/s)  SenseContactSignal=off  NormalStiffness=1e4  NormalStiffnessUnits=N/m  FrictionalCriticalVelocity=1e-3  FrictionalCriticalVelocityUnits=m/s  ZeroCrossDetectContactStartAndEnd=off  SenseContactFollowerRotation=off  SenseContactFollowerTranslation=off  FrictionType=SmoothStickSlip  SenseFrictionalForceMagnitude=off  SenseNormalForceMagnitude=off  NormalForceType=SmoothSpringDamper  SenseNormalVelocity=off  SenseSeparationDistance=off  SenseTangentialVelocity=off  NormalTransitionRegionWidth=1e-3  NormalTransitionRegionWidthUnits=m
  Spatial Contact Force1 : sm_lib/Forces and Torques/Spatial Contact Force  SenseContactBaseRotation=off  SenseContactBaseTranslation=off  CoefficientOfDynamicFriction=0.5  CoefficientOfStaticFriction=0.7  NormalDamping=1e2  NormalDampingUnits=N/(m/s)  SenseContactSignal=off  NormalStiffness=1e4  NormalStiffnessUnits=N/m  FrictionalCriticalVelocity=1e-3  FrictionalCriticalVelocityUnits=m/s  ZeroCrossDetectContactStartAndEnd=off  SenseContactFollowerRotation=off  SenseContactFollowerTranslation=off  FrictionType=SmoothStickSlip  SenseFrictionalForceMagnitude=off  SenseNormalForceMagnitude=off  NormalForceType=SmoothSpringDamper  SenseNormalVelocity=off  SenseSeparationDistance=off  SenseTangentialVelocity=off  NormalTransitionRegionWidth=1e-3  NormalTransitionRegionWidthUnits=m
  Transform Sensor : sm_lib/Frames and Transforms/Transform Sensor  MeasurementFrame=World  SenseAngle=on  SenseAxis=off  SenseAngle1=off  SenseAngle2=off  SenseAngle3=off  SenseQ=off  SenseR=off  SenseOmegaX=off  SenseOmegaY=off  SenseOmegaZ=off  SenseOmega1=off  SenseOmega2=off  SenseOmega3=off  SenseQDot=off  SenseRDot=off  SenseAlphaX=off  SenseAlphaY=off  SenseAlphaZ=off  SenseAlpha1=off  SenseAlpha2=off  SenseAlpha3=off  SenseQDDot=off  SenseRDDot=off  SenseX=off  SenseY=off  SenseZ=off  SenseRad=off  SenseAzim=off  SenseDist=off  SenseInc=off  SenseXDot=off  SenseYDot=off  SenseZDot=off  SenseRadDot=off  SenseAzimDot=off  SenseDistDot=off  SenseIncDot=off  SenseXDDot=off  SenseYDDot=off  SenseZDDot=off  SenseRadDDot=off  SenseAzimDDot=off  SenseDistDDot=off  SenseIncDDot=off
  RP-Bus : PMIOPort  Side=Right
  tag scope: R1motor1q=global, R1motor1w=global, R1motor2q=global, R1motor2w=global, R1tAngle=global, R1tPose=global, R1tRate=global, R1xPose=global, R1yPose=global
  wires:
  [R1motor2t] -> Filter1/1
  [R1motor1t] -> Filter/1(y)
  Gain1/1 -> Simulink-PS Converter1/1
  Gain/1 -> Simulink-PS Converter/1
  Filter/1(x) -> Gain/1
  Filter1/1 -> Gain1/1
  PS-Simulink Converter4/1 -> Interpreted MATLAB Function2/1
  PS-Simulink Converter3/1 -> Interpreted MATLAB Function1/1
  PS-Simulink Converter2/1 -> [R1tPose]  "thetaPose"
  Interpreted MATLAB Function1/1 -> [R1xPose]  "xPose"
  Interpreted MATLAB Function2/1 -> [R1yPose]  "yPose"
  PS-Simulink Converter1/1 -> [R1motor2w]  "motor2w"
  PS-Simulink Converter/1 -> [R1motor2q]  "motor2q"
  PS-Simulink Converter5/1 -> [R1motor1q]  "motor1pose"
  PS-Simulink Converter6/1 -> [R1motor1w]  "motor1w"
  PS-Simulink Converter7/1 -> [R1tRate]
  PS-Simulink Converter8/1 -> [R1tAngle]
  connections:
  Prismatic Joint/RConn1 -- Rigid Transform2/LConn1
  Transform Sensor/RConn1 -- Rigid Transform4/LConn1 -- Planar Joint2/RConn1
  Rigid Transform1/LConn1 -- Rigid Transform/LConn1 -- Sensor Visuals/LConn1 -- Body/LConn1 -- Rigid Transform4/RConn1
  Left Wheel/RConn1 -- Rigid Transform5/LConn1 -- Motor1/RConn1
  Motor2/LConn1 -- Rigid Transform1/RConn1
  Transform Sensor/LConn1 -- Prismatic Joint/LConn1 -- Simscape Bus/LConn3
  Planar Joint2/LConn1 -- Rigid Transform2/RConn1
  Motor1/LConn1 -- Rigid Transform/RConn1
  Rigid Transform3/LConn1 -- Right Wheel/RConn1 -- Motor2/RConn1
  Simulink-PS Converter1/RConn1 -- Motor2/LConn2
  Simulink-PS Converter/RConn1 -- Motor1/LConn2
  Planar Joint2/RConn2 -- PS-Simulink Converter3/LConn1
  Planar Joint2/RConn3 -- PS-Simulink Converter4/LConn1
  Planar Joint2/RConn4 -- PS-Simulink Converter2/LConn1
  Motor1/RConn2 -- PS-Simulink Converter5/LConn1
  Motor1/RConn3 -- PS-Simulink Converter6/LConn1
  PS-Simulink Converter/LConn1 -- Motor2/RConn2
  PS-Simulink Converter1/LConn1 -- Motor2/RConn3
  Rigid Transform3/RConn1 -- Solid/RConn1
  Rigid Transform5/RConn1 -- Solid1/RConn1
  Planar Joint2/RConn5 -- PS-Simulink Converter7/LConn1
  Transform Sensor/RConn2 -- PS-Simulink Converter8/LConn1
  RP-Bus/RConn1 -- Simscape Bus/RConn1
  Spatial Contact Force/RConn1 -- Left Wheel/LConn1
  Simscape Bus/LConn2 -- Spatial Contact Force1/LConn1 -- Spatial Contact Force/LConn1
  Spatial Contact Force1/RConn1 -- Right Wheel/LConn1
  Body/RConn1 -- Simscape Bus/LConn1

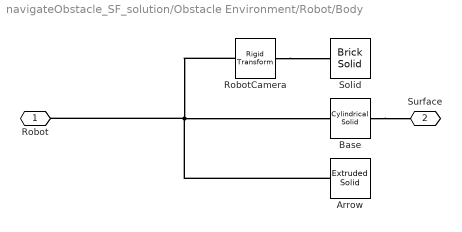
== system navigateObstacle_SF_solution/Obstacle Environment/Robot/Body ==
  Arrow : sm_lib/Body Elements/Extruded Solid  GraphicAmbientColor=[0.15 0.15 0.15 1.0]  BasedOnType=Density  CenterOfMass=[0 0 0]  CenterOfMassUnits=m  GraphicDiffuseColor=[0.8 0.0 1.0]  ExportConvexHullGeometry=off  ExtrusionCrossSection=[1 1; -1 1; -1 -1; 1 -1]  ExtrusionCrossSectionUnits=m  Density=1000  DensityUnits=kg/m^3  DoExposeReferenceFrame=on  GraphicEmissiveColor=[0.0 0.0 0.0 1.0]  ExportEntireGeometry=off  ExtrusionLength=1.3*chassisThickness  ExtrusionLengthUnits=m  ExtrusionType=Regular  SerializedFrames=<Frames/>  MarkerShape=Sphere  MarkerSize=10  GraphicType=FromGeometry  InertiaType=PointMass  Mass=0.2  MassUnits=kg  MomentsOfInertia=[1 1 1]  MomentsOfInertiaUnits=kg*m^2  PolygonNumSides=3  GraphicOpacity=1.0  PolygonOuterRadius=wheelBase/2-wheelBase*0.15  PolygonOuterRadiusUnits=m  ProductsOfInertia=[1 1 1]  ProductsOfInertiaUnits=kg*m^2  GraphicShininess=75  GraphicSpecularColor=[0.5 0.5 0.5 1.0]  GraphicVisPropType=SimpleVisualProperties
  Base : sm_lib/Body Elements/Cylindrical Solid  GraphicAmbientColor=[0.15 0.15 0.15 1.0]  BasedOnType=Mass  CenterOfMass=[0 0 0]  CenterOfMassUnits=m  GraphicDiffuseColor=chassisColor  CylinderLength=chassisThickness  CylinderLengthUnits=m  CylinderRadius=(wheelBase-wheelThickness)/2  CylinderRadiusUnits=m  Density=chassisMass  DensityUnits=kg/m^3  DoExposeReferenceFrame=on  GraphicEmissiveColor=[0.0 0.0 0.0 1.0]  ExportEntireGeometry=on  SerializedFrames=<Frames/>  MarkerShape=Sphere  MarkerSize=10  GraphicType=FromGeometry  InertiaType=CalculateFromGeometry  Mass=chassisMass  MassUnits=kg  MomentsOfInertia=[1 1 1]  MomentsOfInertiaUnits=kg*m^2  GraphicOpacity=1.0  ProductsOfInertia=[1 1 1]  ProductsOfInertiaUnits=kg*m^2  GraphicShininess=75  GraphicSpecularColor=[0.5 0.5 0.5 1.0]  GraphicVisPropType=SimpleVisualProperties
  RobotCamera : sm_lib/Frames and Transforms/Rigid Transform  TranslationMethod=Cartesian  TranslationStandardOffset=0  TranslationLengthUnit=m  TranslationStandardAxis=+Z  TranslationCartesianOffset=[-0.5 0 0.35]  TranslationROffset=0  TranslationROffsetUnits=m  TranslationZOffset=0  TranslationZOffsetUnits=m  TranslationThetaOffset=0  TranslationThetaOffsetUnits=deg  RotationMethod=StandardAxis  RotationAngleUnits=deg  RotationStandardAxis=+Y  RotationAngle=20  RotationArbitraryAxis=[0 0 1]  FollAlignAxisA=+X  BaseAlignAxisA=+Y  FollAlignAxisB=+Y  BaseAlignAxisB=+Z  RotationSequenceAxes=FollowerAxes  RotationSequence=XYX  RotationSequenceAngles=[0 0 0]  RotationSequenceAnglesUnits=deg  RotationMatrix=[1 0 0; 0 1 0; 0 0 1]
  Solid : sm_lib/Body Elements/Brick Solid  GraphicAmbientColor=[0.15 0.15 0.15 1.0]  BasedOnType=Density  BrickDimensions=[0.001 0.001 0.001]  BrickDimensionUnits=m  CenterOfMass=[0 0 0]  CenterOfMassUnits=m  GraphicDiffuseColor=[0.5 0.5 0.5]  Density=1000  DensityUnits=kg/m^3  DoExposeReferenceFrame=on  GraphicEmissiveColor=[0.0 0.0 0.0 1.0]  ExportEntireGeometry=off  SerializedFrames=<Frames/>  MarkerShape=Sphere  MarkerSize=10  GraphicType=FromGeometry  InertiaType=PointMass  Mass=0.00001  MassUnits=kg  MomentsOfInertia=[1 1 1]  MomentsOfInertiaUnits=kg*m^2  GraphicOpacity=0  ProductsOfInertia=[1 1 1]  ProductsOfInertiaUnits=kg*m^2  GraphicShininess=75  GraphicSpecularColor=[0.5 0.5 0.5 1.0]  GraphicVisPropType=SimpleVisualProperties
  Robot : PMIOPort  Side=Left
  Surface : PMIOPort  Port=2  Side=Right
  connections:
  RobotCamera/RConn1 -- Solid/RConn1
  Arrow/RConn1 -- Robot/RConn1 -- RobotCamera/LConn1 -- Base/RConn1
  Base/LConn1 -- Surface/RConn1

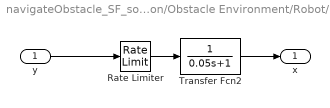
== system navigateObstacle_SF_solution/Obstacle Environment/Robot/Filter ==
  y : Inport
  Rate Limiter : RateLimiter  RisingSlewLimit=300  FallingSlewLimit=-300  SampleTimeMode=inherited
  Transfer Fcn2 : TransferFcn  Denominator=[0.05 1]
  x : Outport  VectorParamsAs1DForOutWhenUnconnected=off
  wires:
  Rate Limiter/1 -> Transfer Fcn2/1
  Transfer Fcn2/1 -> x/1
  y/1 -> Rate Limiter/1

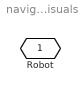
== system navigateObstacle_SF_solution/Obstacle Environment/Robot/Sensor Visuals ==
  Robot : PMIOPort  Side=Left

== stateflow chart navigateObstacle_SF_solution/Navigate Obstacle ==
  state MoveForward
    LeftMotor=100;
    RightMotor=100;
  state TurnLeft
    LeftMotor=-100;
    RightMotor=100;
  (default) -> MoveForward
  MoveForward -> TurnLeft : [after(8,sec)]
  TurnLeft -> MoveForward : [after(2,sec)]
  data: LeftMotor output; RightMotor output
